simulink subsystem "ADC"  (R2023b)
settings: Solver=VariableStepAuto  StartTime=0.0  StopTime=10.0  RelTol=1e-3
libraries: fl_lib x5
settings Model: Creator=torenarginteanu  LastModifiedBy=torenarginteanu

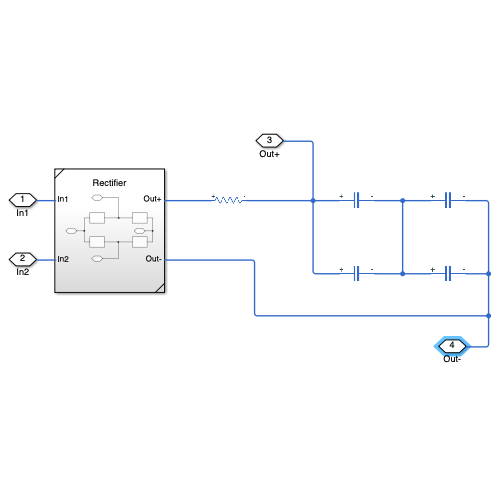
[thumbnail: Simulink's stored preview of the top-level diagram]
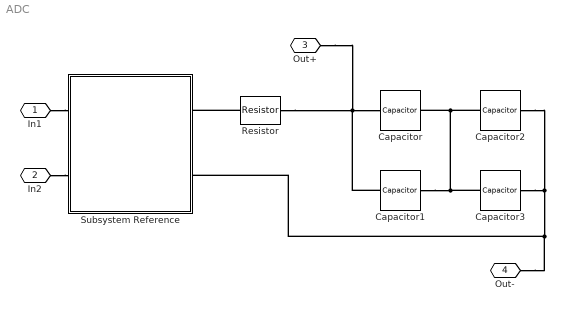
== system ADC ==
  Capacitor{,1..3} (4 alike) : fl_lib/Electrical/Electrical Elements/Capacitor  c=10000 uF  r=1e-6 Ohm  g=0 1/Ohm  i_specify=off  i_priority=None  i=0 A  i_nominal_specify=off  i_nominal_unit=A  i_nominal_value=1  v_specify=off  v_priority=None  v=0 V  v_nominal_specify=off  v_nominal_unit=V  v_nominal_value=1  vc_specify=off  vc_priority=High  vc=0 V  vc_nominal_specify=off  vc_nominal_unit=V  vc_nominal_value=1
  Resistor : fl_lib/Electrical/Electrical Elements/Resistor  R=100 Ohm  i_specify=off  i_priority=None  i=0 A  i_nominal_specify=off  i_nominal_unit=A  i_nominal_value=1  v_specify=off  v_priority=None  v=0 V  v_nominal_specify=off  v_nominal_unit=V  v_nominal_value=1
  Subsystem Reference : Subsystem  ReferencedSubsystem=Rectifier
      settings: PortSchema="{\"entries\":[{\"content\":{\"sides\":[{\"content\":{\"connectorIds\":[\"LConn3\",\"LConn4\"]},\"type\":\"ConnectorPlacement.EquallySpacedRectSide\",\"uuid\":\"0edc6980-720b-4983-80d6-767d37f27a73\"},{\"content\":{\"connectorIds\":[\"LConn2\",\"LConn1\"],\"side\":\"RIGHT\"},\"type\":\"ConnectorPlacement.EquallySpacedRectSide\",\"uuid\":\"c9e36a5a-aeac-4da9-a3a5-158c0c31e496\"},{\"content\":{\"side\":\"TOP\"},\"type\":\"ConnectorPlacement.EquallySpacedRectSide\",\"uuid\":\"9aa74dd9-f64a-4119-8c6d-a301e90ae36e\"}]},\"type\":\"ConnectorPlacement.EquallySpacedConnector\",\"uuid\":\"d44b212d-f1f0-4255-bfdf-751480552c15\"}],\"packageUris\":[\"http://schema.mathworks.com/mf0/Connector/R2020b\"],\"version\":\"1.0\"}"
  In1 : PMIOPort  Side=Left
  In2 : PMIOPort  Port=2  Side=Left
  Out+ : PMIOPort  Port=3  Side=Left
  Out- : PMIOPort  Port=4  Side=Left
  connections:
  In1/RConn1 -- Subsystem Reference/LConn3
  In2/RConn1 -- Subsystem Reference/LConn4
  Resistor/LConn1 -- Subsystem Reference/LConn2
  Capacitor3/LConn1 -- Capacitor1/RConn1 -- Capacitor/RConn1 -- Capacitor2/LConn1
  Resistor/RConn1 -- Capacitor1/LConn1 -- Out+/RConn1 -- Capacitor/LConn1
  Capacitor3/RConn1 -- Out-/RConn1 -- Subsystem Reference/LConn1 -- Capacitor2/RConn1
